simulink library "CEcosimulation"  (Simulink 7.4)
settings: Solver=ode45  StartTime=0.0  StopTime=10.0  RelTol=1e-3
libraries: instrumentlib x2
settings Model: Creator=tasora  LastModifiedBy=tasora

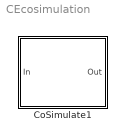
== system CEcosimulation ==
  CoSimulate1 : Subsystem  Description=|  Priority=100  AncestorBlock=CEcosimulation/CoSimulate  mask{com_step=0.001, tcp_data_size=2, host_name=localhost, tcp_port=50009, tcp_timeout=15}
      | This block can be used to exchange data with Chrono.                                                                                             
      | A Chrono program with a running ChCosimulation interface must be started, it will work as a server; then the Simulink program must be run.
      | Note! check that the         dimensions of the exchanged vectors do match!
      mask prompts: com_step "Communication step size"; tcp_data_size "N. of scalars received from C::E (as block output)"; host_name "TCP host name (ex. 'localhost', or 'www.myhost.com')"; tcp_port "TCP port (ex. 50007)"; tcp_timeout "TCP timeout (seconds)"
      mask init:
      | block_receive = [gcb, '/TCP Receive'];
      | set_param(block_receive, 'SampleTime', num2str(com_step));
      | set_param(block_receive, 'Host', host_name);
      | set_param(block_receive, 'Port', num2str(tcp_port));
      | set_param(block_receive, 'DataSize', num2str(tcp_data_size+1));
      | set_param(block_receive, 'Timeout', num2str(tcp_timeout));
      | block_send = [gcb, '/TCP Send'];
      | set_param(block_send, 'Host', host_name);
      | set_param(block_send, 'Port', num2str(tcp_port));
      mask Display:
      | image(imread('block_logo.png'))
      | disp('C::E                   ')

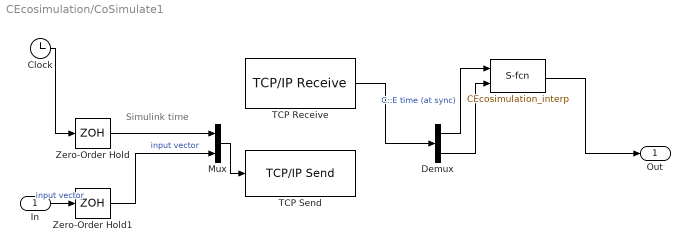
== system CEcosimulation/CoSimulate1 ==
  note: Simulink time
  In : Inport
  " " : M-S-Function  FunctionName=CEcosimulation_interp
  Clock : Clock
      settings: Decimation=10
  Demux : Demux  Outputs=[1 -1]
  Mux : Mux  Inputs=2
  TCP Receive : instrumentlib/TCP//IP Receive  Priority=1  DialogController=instrumentcreatedialog  DialogControllerArgs=DataTag0  Host=localhost  Port=50009  DataSize=3  EnableBlockingMode=on  Timeout=15  SampleTime=0.001  DataType=double  ByteOrder=LittleEndian
  TCP Send : instrumentlib/TCP//IP Send  Priority=2  DialogController=instrumentcreatedialog  DialogControllerArgs=DataTag1  Host=localhost  Port=50009  EnableBlockingMode=on  Timeout=10  ByteOrder=LittleEndian
  Zero-Order Hold : ZeroOrderHold  Priority=0  SampleTime=com_step
  Zero-Order Hold1 : ZeroOrderHold  Priority=0  SampleTime=com_step
  Out : Outport
  wires:
  " "/1 -> Out/1
  Demux/2 -> " "/2
  Demux/1 -> " "/1  "C::E time (at sync)"
  Zero-Order Hold/1 -> Mux/1
  Zero-Order Hold1/1 -> Mux/2  "input vector"
  Mux/1 -> TCP Send/1
  Clock/1 -> Zero-Order Hold/1
  In/1 -> Zero-Order Hold1/1  "input vector"
  TCP Receive/1 -> Demux/1
